simulink subsystem "FineDetune"  (R2024a)
settings: Solver=VariableStepAuto  StartTime=0.0  StopTime=10.0  RelTol=1e-3
settings Model: Creator=dfurodet  LastModifiedBy=david
settings RTWCC: GPUComputeCapability=3.5

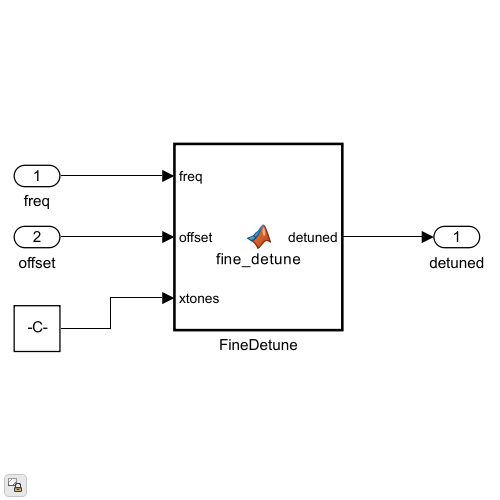
[thumbnail: Simulink's stored preview of the top-level diagram]
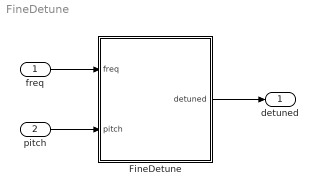
== system FineDetune ==
  freq : Inport
  pitch : Inport  Port=2
  FineDetune : MATLAB Function  Description=|  TreatAsAtomicUnit=on
      | Detunes a frequency in 8th of tones
      | 
      | Which means that an octave is 48 units
  detuned : Outport
  wires:
  pitch/1 -> FineDetune/2(pitch)
  FineDetune/1(detuned) -> detuned/1
  freq/1 -> FineDetune/1(freq)

== matlab function FineDetune/FineDetune ==
  data: freq input; detuned output; pitch input; xtones parameter
function detuned = fine_detune(freq, pitch, xtones)
detuned = power(2, double(pitch) / double(xtones)) * freq;
